simulink model "BUCK_design2"  (R2020b)
settings: Solver=ode23tb  StartTime=0.0  StopTime=0.01  MaxStep=1e-6  RelTol=1e-3
libraries: powerlib x11
settings Model: Creator=91845  LastModifiedBy=91845

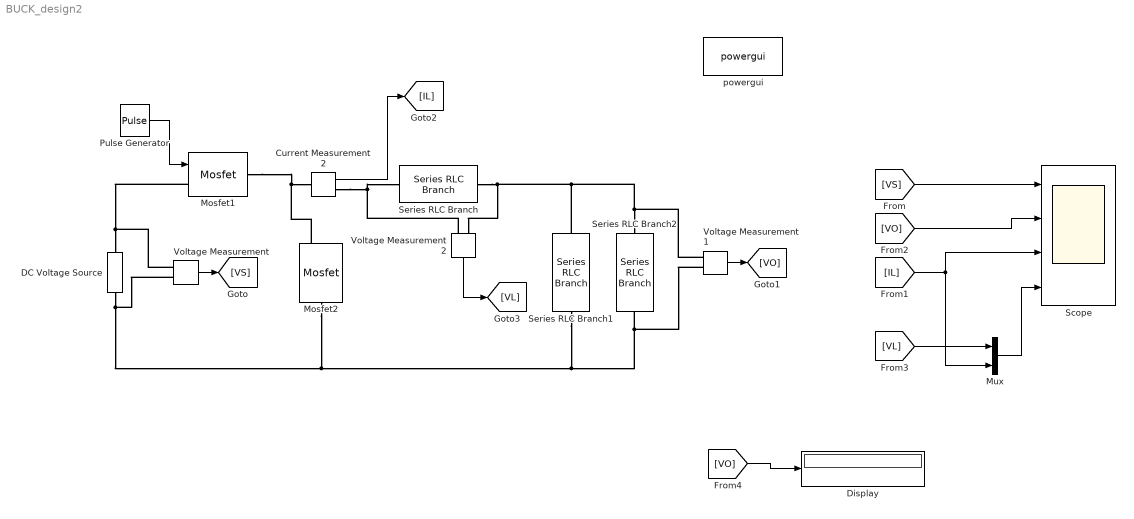
== system BUCK_design2 ==
  Current Measurement2 : powerlib/Measurements/Current Measurement  PhasorSimulation=off  OutputType=Complex  PSBequivalent=0
  DC Voltage Source : powerlib/Electrical Sources/DC Voltage Source  Amplitude=3.3  Measurements=None
  Display : Display
  Mosfet1 : powerlib/Power Electronics/Mosfet  Ron=0  Lon=0  Rd=0  Vfd=0  IC=0  Rs=inf  Cs=inf  Measurements=off
  Mosfet2 : powerlib/Power Electronics/Mosfet  Ron=0  Lon=0  Rd=0  Vfd=0  IC=0  Rs=inf  Cs=inf  Measurements=off
  Mux : Mux  Inputs=2
  Pulse Generator : DiscretePulseGenerator  PulseType=Time based  Period=(1/500e3)  PulseWidth=36.4
  Scope : Scope  NumInputPorts=4
  Series RLC Branch : powerlib/Elements/Series RLC Branch  LConnTagsString=__new0  RConnTagsString=__new0  BranchType=L  Resistance=1  Inductance=1e-6  SetiL0=off  InitialCurrent=0  Capacitance=1e-6  Setx0=off  InitialVoltage=0  Measurements=None
  Series RLC Branch1 : powerlib/Elements/Series RLC Branch  LConnTagsString=__new0  RConnTagsString=__new0  BranchType=RC  Resistance=0.015  Inductance=400e-6  SetiL0=off  InitialCurrent=0  Capacitance=0.16e-6  Setx0=off  InitialVoltage=0  Measurements=None
  Series RLC Branch2 : powerlib/Elements/Series RLC Branch  LConnTagsString=__new0  RConnTagsString=__new0  BranchType=R  Resistance=0.2  Inductance=400e-6  SetiL0=off  InitialCurrent=0  Capacitance=1e-6  Setx0=off  InitialVoltage=0  Measurements=None
  Voltage Measurement : powerlib/Measurements/Voltage Measurement  PhasorSimulation=off  OutputType=Complex  PSBequivalent=0
  Voltage Measurement1 : powerlib/Measurements/Voltage Measurement  PhasorSimulation=off  OutputType=Complex  PSBequivalent=0
  Voltage Measurement2 : powerlib/Measurements/Voltage Measurement  PhasorSimulation=off  OutputType=Complex  PSBequivalent=0
  powergui : powerlib/powergui  Priority=1  SimulationMode=Continuous  SampleTime=50e-6  frequency=60  Iterations=50  frequencyindice=0  Pbase=100e6  ErrMax=1e-4  UnitsV=kV  UnitsW=MW  buscounter=0  FunctionMessages=off  echomessages=off  EnableUseOfTLC=off  CurrentSourceSwitches=off  DisableSnubberDevices=off  DisableRonSwitches=off  DisableVfSwitches=off  DisplayEquations=off  AutomaticDiscreteSolvers=off  SolverType=Tustin/Backward Euler (TBE)  Interpol=off  ExternalGateDelay=off  methode=off  Ts=100  x0status=blocks  SPID=on  SwTol=0  HookPort=off  NonlinearTolerance=1e-4  nMaxIteration=100  ContinueOnMaxIteration=off  RestoreLinks=warning  ResistiveCurrentMeasurement=off  Frange=[0:2:500]  Ylog=off  Xlog=on  ShowGrid=off  save=off  variable=ZData  structure=0  ZoomFFT=off  StartTime=0.0  cycles=1  DisplayStyle=1  fundamental=60  FreqAxis=off  MaxFrequency=1000  frequencyindicesteady=1  RmsSteady=1  display=off
  wires:
  Voltage Measurement/1 -> [VS]
  Voltage Measurement1/1 -> [VO]
  Pulse Generator/1 -> Mosfet1/1
  [VS] -> Scope/1
  [IL] -> Mux/2, Scope/3
  Mux/1 -> Scope/4
  [VO] -> Scope/2
  Voltage Measurement2/1 -> [VL]
  [VL] -> Mux/1
  [VO] -> Display/1
  Current Measurement2/1 -> [IL]
  connections:
  Voltage Measurement/LConn1 -- Mosfet1/LConn1 -- DC Voltage Source/RConn1
  DC Voltage Source/LConn1 -- Voltage Measurement/LConn2 -- Mosfet2/RConn1 -- Series RLC Branch1/LConn1 -- Voltage Measurement1/LConn2 -- Series RLC Branch2/RConn1
  Voltage Measurement2/LConn2 -- Current Measurement2/RConn1 -- Series RLC Branch/LConn1
  Mosfet1/RConn1 -- Mosfet2/LConn1 -- Current Measurement2/LConn1
  Voltage Measurement1/LConn1 -- Series RLC Branch1/RConn1 -- Series RLC Branch/RConn1 -- Voltage Measurement2/LConn1 -- Series RLC Branch2/LConn1
